simulink model "PV_Increment_Conductance_MPPT"  (R2022a)
settings: Solver=ode4  StartTime=0.0  StopTime=10.0  FixedStep=5e-6  RelTol=1e-3
libraries: spsSeriesRLCBranchLib x4, spsVoltageMeasurementLib x2, spsCurrentMeasurementLib x1, spsDiodeLib x1, spsIGBTLib x1, spsPWMGeneratorDCDCLib x1, spsPVArrayLib x1, spspowerguiLib x1
settings Model: Creator=nikos  LastModifiedBy=nikos

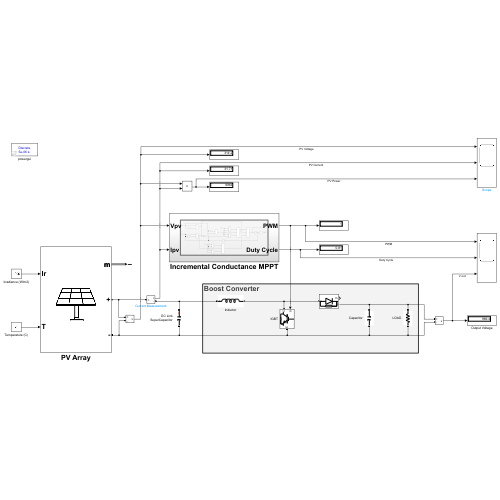
[thumbnail: Simulink's stored preview of the top-level diagram]
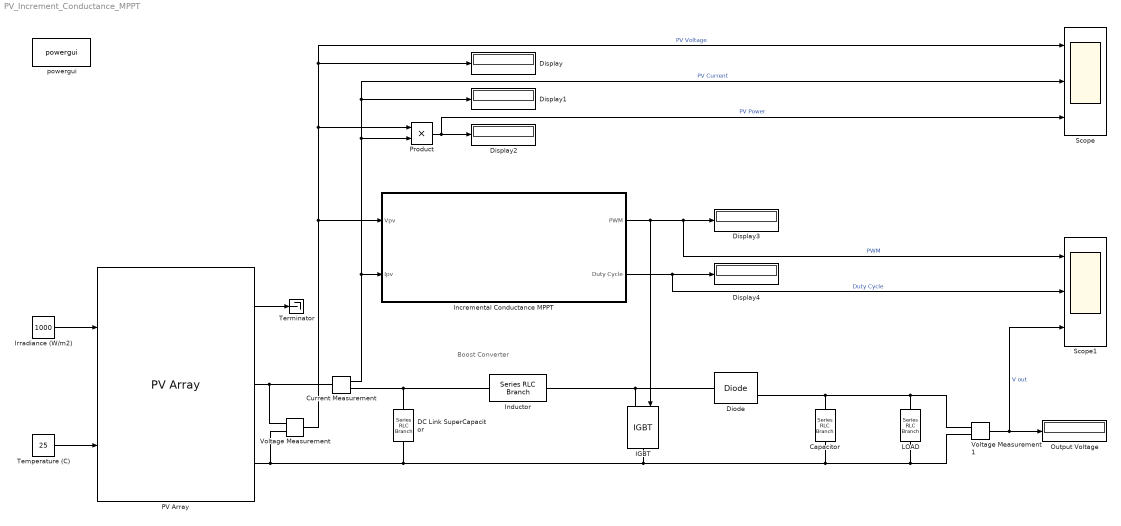
== system PV_Increment_Conductance_MPPT ==
  note: Boost Converter
  Capacitor : spsSeriesRLCBranchLib/Series RLC Branch  LConnTagsString=__new0  RConnTagsString=__new0  BranchType=C  Resistance=1  Inductance=1e-3  SetiL0=off  InitialCurrent=0  Capacitance=5e-3  Setx0=off  InitialVoltage=0  Measurements=None
  Current Measurement : spsCurrentMeasurementLib/Current Measurement  PhasorSimulation=off  OutputType=Complex  PSBequivalent=0
  DC Link SuperCapacitor : spsSeriesRLCBranchLib/Series RLC Branch  LConnTagsString=__new0  RConnTagsString=__new0  BranchType=C  Resistance=1  Inductance=1e-3  SetiL0=off  InitialCurrent=0  Capacitance=3e-3  Setx0=off  InitialVoltage=0  Measurements=None
  Diode : spsDiodeLib/Diode  Ron=0.001  Lon=0  Vf=0.8  IC=0  UseSnubber=0  Rs=500  Cs=250e-9  Measurements=on
  Display{,1..4} (5 alike) : Display
  IGBT : spsIGBTLib/IGBT  Ron=0.001  Lon=0  Vf=1  Tf=1e-6  Tt=2e-6  IC=0  Rs=1e5  Cs=inf  Measurements=off
  Incremental Conductance MPPT : Subsystem
  Inductor : spsSeriesRLCBranchLib/Series RLC Branch  LConnTagsString=__new0  RConnTagsString=__new0  BranchType=L  Resistance=1  Inductance=1e-3  SetiL0=off  InitialCurrent=0  Capacitance=1e-6  Setx0=off  InitialVoltage=0  Measurements=None
  Irradiance (W/m2) : Constant  Value=1000
  LOAD : spsSeriesRLCBranchLib/Series RLC Branch  LConnTagsString=__new0  RConnTagsString=__new0  BranchType=R  Resistance=100  Inductance=1e-3  SetiL0=off  InitialCurrent=0  Capacitance=1e-6  Setx0=off  InitialVoltage=0  Measurements=None
  Output Voltage : Display
  PV Array : spsPVArrayLib/PV Array  Npar=4  Nser=10  PlotType=array @ 1000 W/m2 & specified temperatures  S_vec="[ 1000  500  100 ]"  Temp_C_vec="[ 25  ]"  ModuleName=User-defined  PlotWhenSelected=off  Pm=249.86  Ncell=60  Voc=37.6  Isc=8.55  Vm=31  Im=8.06  beta_Voc_pc=-0.35  alpha_Isc_pc=0.06  beta_Voc=-0.1316  alpha_Isc=0.00513  IL=8.5795  I0=2.0381e-10  nI=0.99766  Rsh=301.8149  Rs=0.247  RobustModel=off  RobustCellTemperature=313.3991  BAL=on  Tc=1e-6  Tfilter=5e-5
  Product : Product
  Scope : Scope  NumInputPorts=3
  Scope1 : Scope  NumInputPorts=3
  Temperature (C) : Constant  Value=25
  Terminator : Terminator
  Voltage Measurement : spsVoltageMeasurementLib/Voltage Measurement  PhasorSimulation=off  OutputType=Complex  PSBequivalent=0
  Voltage Measurement1 : spsVoltageMeasurementLib/Voltage Measurement  PhasorSimulation=off  OutputType=Complex  PSBequivalent=0
  powergui : spspowerguiLib/powergui  Priority=1  SimulationMode=Discrete  SampleTime=5e-6  frequency=60  Iterations=50  frequencyindice=0  Pbase=100e6  ErrMax=1e-4  UnitsV=kV  UnitsW=MW  buscounter=0  FunctionMessages=off  echomessages=off  EnableUseOfTLC=off  CurrentSourceSwitches=off  DisableSnubberDevices=off  DisableRonSwitches=off  DisableVfSwitches=off  DisplayEquations=off  AutomaticDiscreteSolvers=off  SolverType=Tustin/Backward Euler (TBE)  Interpol=off  ExternalGateDelay=off  methode=off  Ts=100  x0status=blocks  SPID=on  SwTol=0  HookPort=off  NonlinearTolerance=1e-4  nMaxIteration=100  ContinueOnMaxIteration=off  RestoreLinks=warning  ResistiveCurrentMeasurement=off  Frange=[0:2:500]  Ylog=off  Xlog=on  ShowGrid=off  save=off  variable=ZData  structure=0  ZoomFFT=off  StartTime=0.0  cycles=1  DisplayStyle=1  fundamental=60  FreqAxis=off  MaxFrequency=1000  frequencyindicesteady=1  RmsSteady=1  display=off
  wires:
  Irradiance (W/m2)/1 -> PV Array/1
  Temperature (C)/1 -> PV Array/2
  PV Array/1 -> Terminator/1
  Product/1 -> Scope/3, Display2/1  "PV Power"
  Voltage Measurement/1 -> Scope/1, Display/1, Product/1, Incremental Conductance MPPT/1(Vpv)  "PV Voltage"
  Current Measurement/1 -> Product/2, Display1/1, Scope/2, Incremental Conductance MPPT/2(Ipv)  "PV Current"
  Incremental Conductance MPPT/1(PWM) -> Scope1/1, Display3/1, IGBT/1  "PWM"
  Voltage Measurement1/1 -> Scope1/3, Output Voltage/1  "V out"
  Incremental Conductance MPPT/2(Duty Cycle) -> Scope1/2, Display4/1  "Duty Cycle"
  connections:
  DC Link SuperCapacitor/LConn1 -- Inductor/LConn1 -- Current Measurement/RConn1
  DC Link SuperCapacitor/RConn1 -- Voltage Measurement1/LConn2 -- LOAD/RConn1 -- Capacitor/RConn1 -- IGBT/RConn1 -- Voltage Measurement/LConn2 -- PV Array/RConn2
  IGBT/LConn1 -- Diode/LConn1 -- Inductor/RConn1
  Capacitor/LConn1 -- Voltage Measurement1/LConn1 -- LOAD/LConn1 -- Diode/RConn1
  Current Measurement/LConn1 -- Voltage Measurement/LConn1 -- PV Array/RConn1

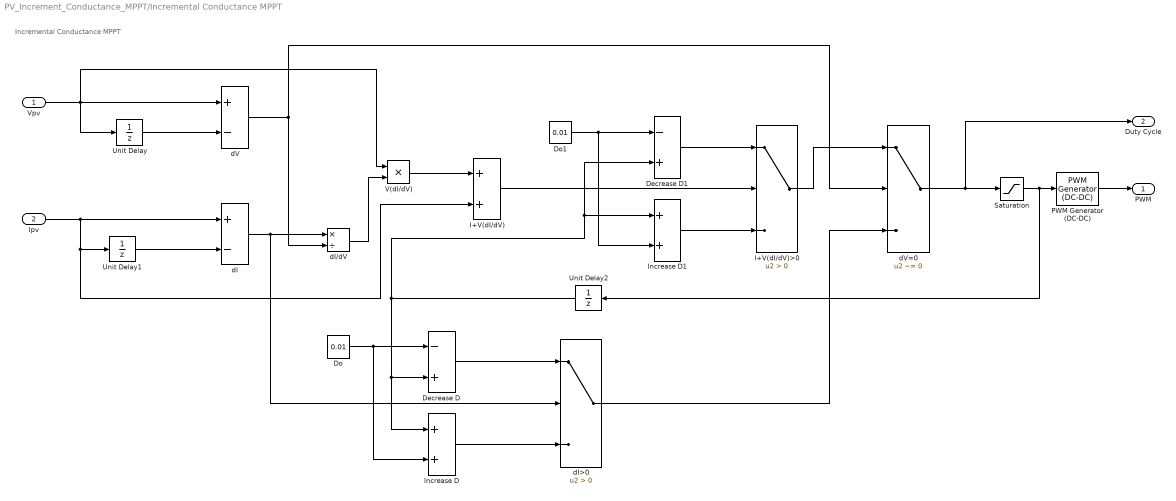
== system PV_Increment_Conductance_MPPT/Incremental Conductance MPPT ==
  note: Incremental Conductance MPPT
  Vpv : Inport
  Ipv : Inport  Port=2
  Decrease D : Sum  Inputs=-+
  Decrease D1 : Sum  Inputs=-+
  Do : Constant  Value=0.01
  Do1 : Constant  Value=0.01
  I+V(dI/dV) : Sum
  I+V(dI/dV)>0 : Switch  Criteria=u2 > Threshold  SaturateOnIntegerOverflow=off  InputSameDT=off
  Increase D : Sum
  Increase D1 : Sum
  PWM Generator (DC-DC) : spsPWMGeneratorDCDCLib/PWM Generator (DC-DC)  Fsw=1000  Ts=5e-6
  Saturation : Saturate  UpperLimit=0.8  LowerLimit=0.1
  Unit Delay : UnitDelay  SampleTime=5e-6  HasFrameUpgradeWarning=on
  Unit Delay1 : UnitDelay  SampleTime=5e-6  HasFrameUpgradeWarning=on
  Unit Delay2 : UnitDelay  SampleTime=5e-6  HasFrameUpgradeWarning=on
  V(dI/dV) : Product
  dI : Sum  Inputs=+-
  dI/dV : Product  Inputs=*/
  dI>0 : Switch  Criteria=u2 > Threshold  SaturateOnIntegerOverflow=off  InputSameDT=off
  dV : Sum  Inputs=+-
  dV=0 : Switch  Criteria=u2 ~= 0  SaturateOnIntegerOverflow=off  InputSameDT=off
  PWM : Outport
  Duty Cycle : Outport  Port=2
  wires:
  Vpv/1 -> Unit Delay/1, V(dI/dV)/1, dV/1
  Ipv/1 -> Unit Delay1/1, I+V(dI/dV)/2, dI/1
  Unit Delay/1 -> dV/2
  Unit Delay1/1 -> dI/2
  dI/1 -> dI>0/2, dI/dV/1
  dV/1 -> dV=0/2, dI/dV/2
  dI/dV/1 -> V(dI/dV)/2
  V(dI/dV)/1 -> I+V(dI/dV)/1
  Do/1 -> Increase D/2, Decrease D/1
  Unit Delay2/1 -> Increase D/1, Decrease D/2, Decrease D1/2, Increase D1/1
  Decrease D/1 -> dI>0/1
  Increase D/1 -> dI>0/3
  Do1/1 -> Increase D1/2, Decrease D1/1
  I+V(dI/dV)/1 -> I+V(dI/dV)>0/2
  Decrease D1/1 -> I+V(dI/dV)>0/1
  Increase D1/1 -> I+V(dI/dV)>0/3
  I+V(dI/dV)>0/1 -> dV=0/1
  dI>0/1 -> dV=0/3
  dV=0/1 -> Duty Cycle/1, Saturation/1
  PWM Generator (DC-DC)/1 -> PWM/1
  Saturation/1 -> Unit Delay2/1, PWM Generator (DC-DC)/1
